simulink model "translationalkinematicsii"  (R2023a)
settings: Solver=VariableStepAuto  StartTime=0.0  StopTime=1000.0  RelTol=1e-3
undefined symbols (not defined in the file): x0
libraries: matrix_library x2
settings Model: Creator=prafulsigdel  LastModifiedBy=prafulsigdel

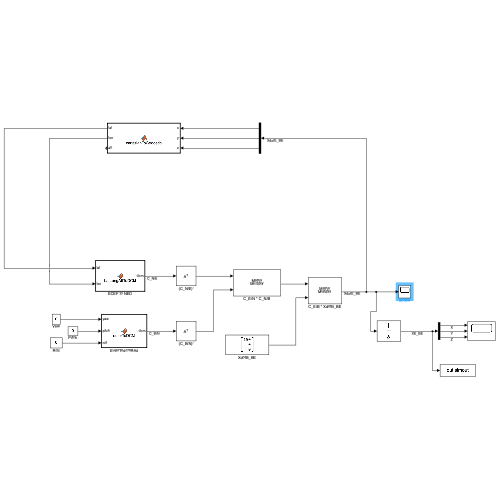
[thumbnail: Simulink's stored preview of the top-level diagram]
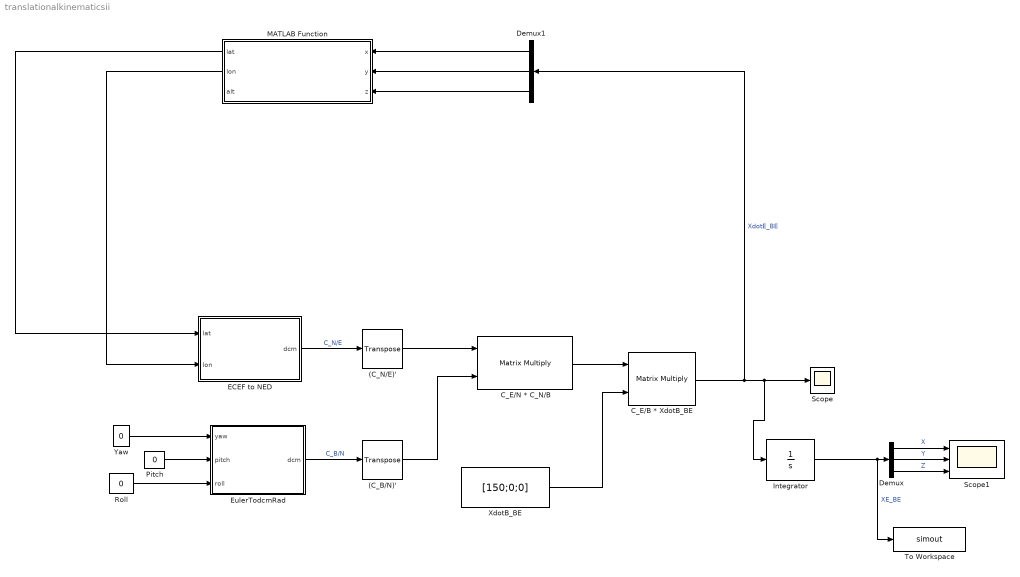
== system translationalkinematicsii ==
  (C_B/N)' : matrix_library/Transpose
  (C_N/E)' : matrix_library/Transpose
  C_E/B * XdotB_BE : Product  Multiplication=Matrix(*)
  C_E/N * C_N/B : Product  Multiplication=Matrix(*)
  Demux : Demux  Outputs=3
  Demux1 : Demux  Outputs=3
  ECEF to NED : MATLAB Function  TreatAsAtomicUnit=on
  EulerTodcmRad : MATLAB Function  TreatAsAtomicUnit=on
  Integrator : Integrator  InitialCondition=x0
  MATLAB Function : MATLAB Function  TreatAsAtomicUnit=on
  Pitch : Constant  Value=0
  Roll : Constant  Value=0
  Scope : Scope
  Scope1 : Scope  NumInputPorts=3
  To Workspace : ToWorkspace  VariableName=simout  SaveFormat=Timeseries  SampleTime=-1
  XdotB_BE : Constant  Value=[150;0;0]  VectorParams1D=off
  Yaw : Constant  Value=0
  wires:
  Demux1/2 -> MATLAB Function/2(y)
  Demux1/1 -> MATLAB Function/1(x)
  C_E/B * XdotB_BE/1 -> Demux1/1, Integrator/1, Scope/1  "XdotE_BE"
  Demux1/3 -> MATLAB Function/3(z)
  Demux/2 -> Scope1/2  "Y"
  (C_B/N)'/1 -> C_E/N * C_N/B/2
  ECEF to NED/1(dcm) -> (C_N/E)'/1  "C_N/E"
  Pitch/1 -> EulerTodcmRad/2(pitch)
  Demux/3 -> Scope1/3  "Z"
  Integrator/1 -> To Workspace/1, Demux/1  "XE_BE"
  Demux/1 -> Scope1/1  "X"
  EulerTodcmRad/1(dcm) -> (C_B/N)'/1  "C_B/N"
  C_E/N * C_N/B/1 -> C_E/B * XdotB_BE/1
  Roll/1 -> EulerTodcmRad/3(roll)
  XdotB_BE/1 -> C_E/B * XdotB_BE/2
  Yaw/1 -> EulerTodcmRad/1(yaw)
  (C_N/E)'/1 -> C_E/N * C_N/B/1
  MATLAB Function/1(lat) -> ECEF to NED/1(lat)
  MATLAB Function/2(lon) -> ECEF to NED/2(lon)

== matlab function translationalkinematicsii/ECEF to NED ==
  data: lat input; dcm output; lon input
function dcm = LatLongAttToDCM(lat, lon)
% Convert euler angles to DCM
C_NE = [0 0 1; 0 1 0; -1 0 0];
C_NdN = [cos(lat) 0 sin(lat); 0 1 0; -sin(lat) 0 cos(lat)];
C_NNd = [1 0 0; 0 cos(lon) -sin(lon); 0 sin(lon) cos(lon)];

% Convert DCM
dcm = C_NNd * C_NdN * C_NE;

end

== matlab function translationalkinematicsii/EulerTodcmRad ==
  data: yaw input; dcm output; pitch input; roll input
function dcm = eulerToDCM(yaw, pitch, roll)
% Convert euler angles to DCM angles in Radians.
C_Y = [cos(yaw) -sin(yaw) 0; sin(yaw) cos(yaw) 0;0 0 1];
C_P = [cos(pitch) 0 sin(pitch); 0 1 0; -sin(pitch) 0 cos(pitch)];
C_R = [1 0 0; 0 cos(roll) -sin(roll); 0 sin(roll) cos(roll)];

% Convert DCM
dcm = C_R * C_P * C_Y;

end

== matlab function translationalkinematicsii/MATLAB Function ==
  data: x input; lat output; y input; z input; lon output; alt output
function [lat, lon, alt] = cartesianToGeodetic(x, y, z)

    % WGS84 ellipsoid parameters
    a = 6378137;     % Semi-major axis (meters)
    f = 1/298.257223563;  % Flattening
    b = a * (1 - f); % Semi-minor axis (meters)

    % Eccentricity squared
    e2 = (a^2 - b^2) / a^2;

    % Calculate longitude
    lon = atan2(y, x);

    % Calculate latitude
    p = sqrt(x^2 + y^2);
    theta = atan2(z * a, p * b);
    lat = atan2(z + e2 * b * sin(theta)^3, p - e2 * a * cos(theta)^3);

    % Calculate altitude
    N = a / sqrt(1 - e2 * sin(lat)^2);
    alt = p / cos(lat) - N;

end
